simulink model "Inverter"  (Simulink 8.6)
settings: Solver=ode45  StartTime=0.0  StopTime=12000  FixedStep=0.02  RelTol=1e-6
settings Model: Creator=Yi  LastModifiedBy=DAZE
settings SolverCC: ZeroCrossAlgorithm=Adaptive
settings DebuggingCC: MaxConsecutiveZCsMsg=none  FcnCallInpInsideContextMsg=EnableAllAsWarning
settings GRTTargetCC: CombineOutputUpdateFcns=on  GRTInterface=off

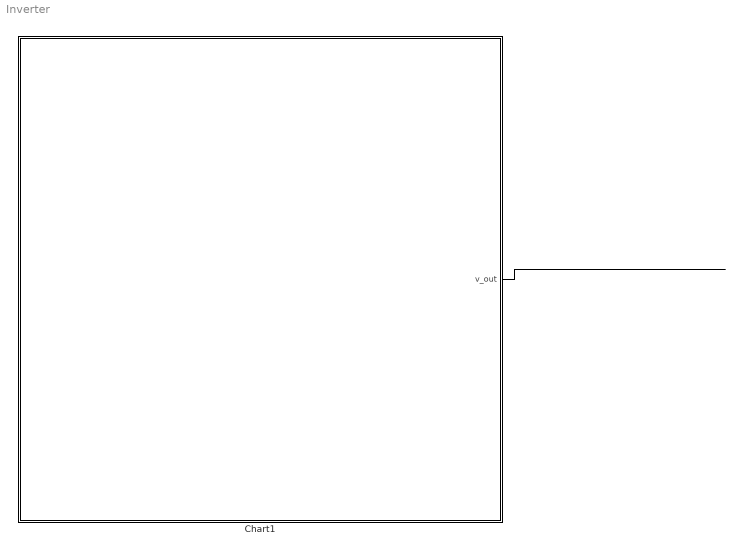
== system Inverter ==
  Chart1 : Stateflow chart  TreatAsAtomicUnit=on
  wires:
  Chart1/1(v_out) -> ?

== stateflow chart Chart1 ==
  settings: updateMethod=CONTINUOUS
  state C
    du:
    v_dot=((0.000519/2)*(1.2-vin-0.47)*(1.2-vin-0.47))*1000000;
    vin_dot = 0;
    v_out=v;
  state A
    du:
    v_dot=(0.000519 * (1.2 - v) * (1.2 - vin - 0.47 - (1.2-v)/2))*1000000;
    vin_dot = 0;
    v_out=v;
  state B
    du:
    v_dot=(0.000519 * (1.2 - v) * (1.2-vin-0.47-(1.2-v)/2) - (0.000459/2) * (vin-0.4)*(vin-0.4))*1000000;
    vin_dot = 0;
    v_out=v;
  state D
    du:
    v_dot=((0.000519/2)*(1.2-vin-0.47)*(1.2-vin-0.47) - (0.000459/2)*(vin-0.4)*(vin-0.4))*1000000;
    vin_dot = 0;
    v_out=v;
  state E
    du:
    v_dot=((0.000519/2)*(1.2-vin-0.47)*(1.2-vin-0.47) - (0.000459*v)*(vin-0.4-(v/2)))*1000000;
    vin_dot = 0;
    v_out=v;
  state F
    du:
    v_dot=(-0.000459 * (vin - 0.4)*(vin - 0.4))*1000000;
    vin_dot = 0;
    v_out=v;
  state G
    du:
    v_dot=(-0.000459 * v * (vin - 0.4 - (v/2)))*1000000;
    vin_dot = 0;
    v_out=v;
  G -> F : [vin<0.73]
  E -> G [order 2] : [vin>0.73]
  F -> G [order 2] : [vin>0.73]
  F -> D [order 1] : [vin<0.73]
  D -> F [order 3] : [vin>0.73]
  E -> D [order 1] : [vin<v+0.4]
  D -> E [order 4] : [vin>v+0.4]
  D -> B [order 1] : [vin<v-0.47]
  C -> D [order 2] : [vin>0.4]
  D -> C [order 2] : [vin<0.4]
  B -> D [order 2] : [vin>v-0.47]
  C -> A [order 1] : [vin<v - 0.47]
  A -> B : [vin>0.4]
  B -> A [order 1] : [vin<0.4]
  (default) -> A : {vin=0,v=0}
  data: v local double; v_out output double; vin local double =0
  data v settings: updateMethod=SF_CONTINUOUS_TIME_DATA
  data vin settings: updateMethod=SF_CONTINUOUS_TIME_DATA
